simulink model "CPS_heave_noAccelmeter_20221201"  (R2022b)
settings: Solver=ode4  StartTime=0.0  StopTime=sim_time  RelTol=1e-3  EnableMultiTasking=on
values from neighbouring files (symbols this model uses):
  c = 2*dampratio*sqrt(k*M)    [CPS_sims_and_analysis.m]    (also in command_limits_check.m; ringdown-circcyl-M10-d0_001-F1-workspace.mat = 0.125663706144; setup_CPS_parameters.m)
  k = (2*pi*f_nat)^2*M    (= 394.784176044)    [CPS_sims_and_analysis.m]    (also in command_limits_check.m = 98.6960440109; ringdown-circcyl-M10-d0_001-F1-workspace.mat; setup_CPS_parameters.m)
  M = 10    [CPS_sims_and_analysis.m]    (also in command_limits_check.m; ringdown-circcyl-M10-d0_001-F1-workspace.mat; setup_CPS_parameters.m)
  start_position_meters = last_out(6)*-0.03    [CPS_heave_move_2_setpoint.m]
  T = 0.0002    [ringdown-circcyl-M10-d0_001-F1-workspace.mat]    (also in setup_CPS_parameters.m = 0.001)
  Wallace_Cal_tranp = [-0.14949 0.21629 -0.44045 -69.17754 5.14209 66.58631 3.76511 79.12451 -0.93703 -39.93894 -3.18235 -38.82968 ... (36 elements, 6x6)]    [ringdown-circcyl-M10-d0_001-F1-workspace.mat]    (also in setup_CPS_parameters.m = Wallace_Cal')
undefined symbols (not defined in the file or in its folder): DiscIntNeverNeededParam, National_Instruments, PCIe, sigbuilder_block
libraries: sldrtlib x5, dsparch4 x1
settings Model: SimulationMode=external  ExtModeTrigDuration=8000000  Creator=Control Systems  LastModifiedBy=eericks1
settings SolverCC: AlgebraicLoopSolver=TrustRegion
settings DataIOCC: MaxDataPoints=10000  SaveFormat=StructureWithTime  ReturnWorkspaceOutputs=off
settings DebuggingCC: UnconnectedInputMsg=warning  UnconnectedOutputMsg=warning  UnconnectedLineMsg=warning  SFUnexpectedBacktrackingDiag=warning  SFNoUnconditionalDefaultTransitionDiag=warning  SFExecutionAtInitializationDiag=none  SFMachineParentedDataDiag=warning  ArithmeticOperatorsInVariantConditions=warning
settings HardwareCC: ProdBitPerLong=64  ProdHWDeviceType=Intel->x86-64 (Linux 64)  TargetBitPerLong=64  TargetBitPerPointer=64  TargetIntDivRoundTo=Zero  TargetEndianess=LittleEndian  TargetWordSize=64  TargetHWDeviceType=Intel->x86-64
settings ModelReferenceCC: EnableRefExpFcnMdlSchedulingChecks=on  PropagateSignalLabelsOutOfModel=off
settings SFSimCC: SimUseLocalCustomCode=off  CustomCodeUndefinedFunction=UseInterfaceOnly
settings RTWCC: Description=Simulink Desktop Real-Time  SystemTargetFile=sldrt.tlc  TemplateMakefile=sldrt.tmf  RTWUseLocalCustomCode=off  RTWCompilerOptimization=on
settings CodeAppCC: MaxIdLength=95  StateflowObjectComments=on
settings SimulinkDesktopRealTimeCC: TargetLibSuffix=_sldrt.a  TargetPreCompLibLocation=C:\Program Files\MATLAB\R2022b\toolbox\sldrt\lib\win64  TargetLangStandard=C89/C90 (ANSI)  SupportVariableSizeSignals=off
settings ConfigComp: CovMetricSettings=dw  CovSaveCumulativeToWorkspaceVar=on  CovSaveSingleToWorkspaceVar=on  CovExternalEMLEnable=off

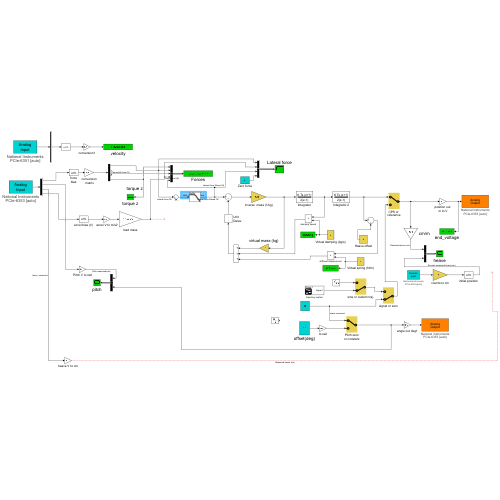
[thumbnail: Simulink's stored preview of the top-level diagram]
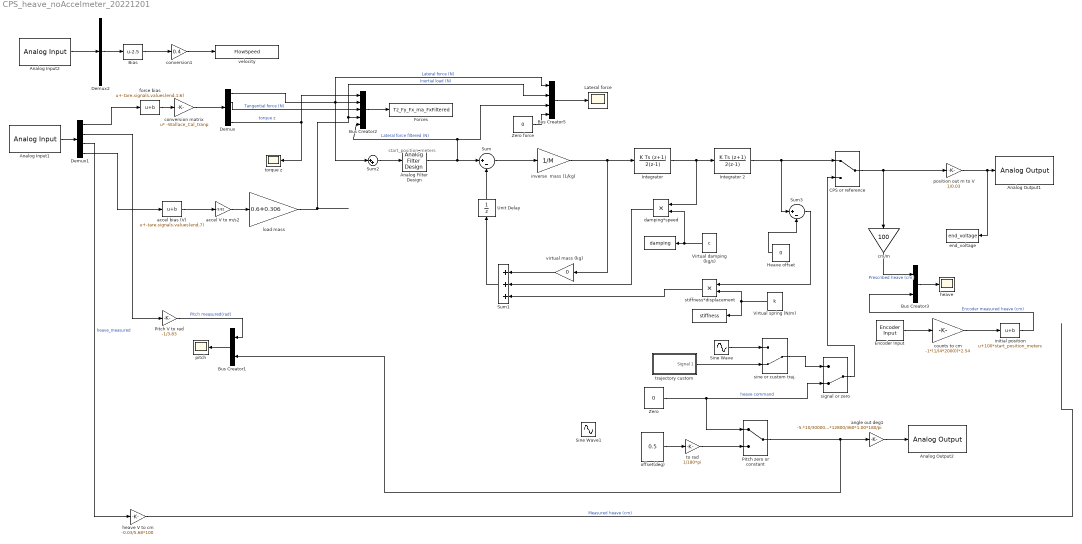
== system CPS_heave_noAccelmeter_20221201 ==
  note: start_position_meters
  " " : ToWorkspace  VariableName=damping  SaveFormat=Structure With Time  SampleTime=-1
  "  " : ToWorkspace  VariableName=stiffness  SaveFormat=Structure With Time  SampleTime=-1
  Analog Filter Design : dsparch4/Analog Filter Design  method=Butterworth  filttype=Lowpass  N=4  Wlo=2*3.14*10  Whi=80  Rp=2  Rs=40
  Analog Input1 : sldrtlib/Analog Input  SampleTime=T  MaxMissedTicks=10  ShowMissedTicks=off  YieldWhenWaiting=off  DrvName=National_Instruments/PCIe-6353  DrvAddress=4294967295  DrvOptions=[0 0 0 2 2 2 2]  Channels=[1: 6 23 24 25]  RangeMode=1  VoltRange=1  DataType=1
      settings: AttributesFormatString=National Instruments\nPCIe-6353 [auto]
  Analog Input2 : sldrtlib/Analog Input  SampleTime=T  MaxMissedTicks=10  ShowMissedTicks=off  YieldWhenWaiting=off  DrvName=National_Instruments/PCIe-6351  DrvAddress=4294967295  DrvOptions=[0 0 0 0 0 0 0]  Channels=[7:10]  RangeMode=1  VoltRange=1  DataType=1
      settings: AttributesFormatString=National Instruments\nPCIe-6351 [auto]
  Analog Output1 : sldrtlib/Analog Output  SampleTime=T  MaxMissedTicks=10  ShowMissedTicks=off  YieldWhenWaiting=off  DrvName=National_Instruments/PCIe-6353  DrvAddress=4294967295  DrvOptions=[0 0 0 2 2 2 2]  Channels=[2]  RangeMode=1  VoltRange=1  InitialValue=[]  FinalValue=[]
      settings: AttributesFormatString=National Instruments\nPCIe-6353 [auto]
  Analog Output2 : sldrtlib/Analog Output  SampleTime=T  MaxMissedTicks=10  ShowMissedTicks=off  YieldWhenWaiting=off  DrvName=National_Instruments/PCIe-6353  DrvAddress=4294967295  DrvOptions=[0 0 0 2 2 2 2]  Channels=[1]  RangeMode=1  VoltRange=1  InitialValue=[]  FinalValue=[]
      settings: AttributesFormatString=National Instruments\nPCIe-6353 [auto]
  Bias : Bias  Bias=-2.5  SaturateOnIntegerOverflow=off
  Bus Creator1 : BusCreator  Inputs=2
  Bus Creator2 : BusCreator  Inputs=5
  Bus Creator3 : BusCreator  Inputs=2
  Bus Creator5 : BusCreator  Inputs=4
  CPS or reference : ManualSwitch
  Demux : Demux  Outputs=[1 1 3 1]
  Demux1 : Demux  Outputs=[6 1 1 1]
  Demux2 : Demux  Outputs=[4]
  Encoder Input : sldrtlib/Encoder Input  SampleTime=T  MaxMissedTicks=10  ShowMissedTicks=off  YieldWhenWaiting=off  DrvName=National_Instruments/PCIe-6353  DrvAddress=4294967295  DrvOptions=[0 0 0 2 2 2 2]  Channels=[1]  QuadMode=3  IndexPulse=1  InputFilter=Inf  DataType=1
      settings: AttributesFormatString=National Instruments\nPCIe-6353 [auto]
  Forces : ToWorkspace  VariableName=Tz_Fy_Fx_ma_FxFiltered  SaveFormat=Structure With Time  SampleTime=-1
  Heave offset : Constant  Value=0  SampleTime=T
  Integrator : DiscreteIntegrator  IntegratorMethod=Integration: Trapezoidal  SampleTime=-1  ICPrevOutput=DiscIntNeverNeededParam  ICPrevScaledInput=DiscIntNeverNeededParam
  Integrator 2 : DiscreteIntegrator  IntegratorMethod=Integration: Trapezoidal  InitialCondition=start_position_meters  SampleTime=-1  ICPrevOutput=DiscIntNeverNeededParam  ICPrevScaledInput=DiscIntNeverNeededParam
  Lateral force : Scope
  Pitch V to rad : Gain  Gain=-1/3.83
  Pitch zero or constant : ManualSwitch
  Sine Wave : Sin  Amplitude=0.05  Frequency=2*3.14*1  SampleTime=0
  Sine Wave1 : Sin  Frequency=2*3.14*0.5  SampleTime=0
  Sum : Sum  Inputs=|+-
  Sum1 : Sum  Inputs=+++
  Sum2 : Sum  Inputs=|++
  Sum3 : Sum  Inputs=|+-
  Unit Delay : UnitDelay  InitialCondition=-start_position_meters*k/M  SampleTime=-1  HasFrameUpgradeWarning=on
  Virtual damping (kg/s) : Constant  Value=c  SampleTime=T
  Virtual spring (N/m) : Constant  Value=k  SampleTime=T
  Zero : Constant  Value=0  SampleTime=T
  Zero force : Constant  Value=0  SampleTime=T
  accel V to m/s2 : Gain  Gain=-9.81
  accel bias (V) : Bias  Bias=-tare.signals.values(end,7)  SaturateOnIntegerOverflow=off
  angle out deg1 : Gain  Gain=-5.*10/30000*12800/360*1.00*180/pi
  cm/m : Gain  Gain=100
  conversion matrix : Gain  Gain=-Wallace_Cal_tranp  Multiplication=Matrix(u*K)
  conversion1 : Gain  Gain=0.4
  counts to cm : Gain  Gain=-1*(1/(4*2000))*2.54
  damping*speed : Product
  end_voltage : ToWorkspace  VariableName=end_voltage  SampleTime=-1
      settings: MaxDataPoints=1
  force bias : Bias  Bias=-tare.signals.values(end,1:6)  SaturateOnIntegerOverflow=off
  heave : Scope
  heave V to cm : Gain  Gain=-0.03/5.68*100
  initial position : Bias  Bias=100*start_position_meters  SaturateOnIntegerOverflow=off
  "inverse  mass (1/kg) " : Gain  Gain=1/M
  load mass : Gain  Gain=0.6+0.306
  offset(deg) : Constant  Value=0.5  SampleTime=T
  pitch : Scope
  position out m to V : Gain  Gain=1/0.03
  signal or zero : ManualSwitch  CurrentSetting=0
  sine or custom traj. : ManualSwitch  CurrentSetting=0
  stiffness*displacement : Product
  to rad : Gain  Gain=1/180*pi
  torque z : Scope
  trajectory custom : Subsystem  Tag=STV Subsys  LoadFcn=sigbuilder_block('load');  StartFcn=sigbuilder_block('start');  StopFcn=sigbuilder_block('stop');  ClipboardFcn=sigbuilder_block('clipboard');  mask(Sigbuilder block){tuvar=[0:10]}
      mask help: Simulink:masks:SigbuilderBlock_MD
      mask init:
      | if ~strcmp(get_param(bdroot(gcbh),'SimulationStatus'),'stopped') tuvar = sigbuilder_block('maskInit'); end
      settings: CopyFcn=sigbuilder_block('copy');  DeleteFcn=sigbuilder_block('delete');  ModelCloseFcn=sigbuilder_block('modelClose');  PreSaveFcn=sigbuilder_block('preSave');  PauseFcn=sigbuilder_block('pause');  ContinueFcn=sigbuilder_block('continue');  NameChangeFcn=sigbuilder_block('namechange');  OpenFcn=sigbuilder_block('open',[270 192.75 550.5 399.75 ]);  CloseFcn=sigbuilder_block('close');
      mask Display: plot(0, 0, 100, 100,[2, 2, 32, 32, 2], [68, 8, 8, 68, 68],[32, 2], [38, 38], [32, 19, 2],[53, 60, 44], [32, 17, 17, 2],[16, 16, 31, 31]);txt = getActiveGroup(gcbh);text(2, 100, txt,'verticalAlignment', 'top');
  velocity : ToWorkspace  VariableName=FlowSpeed  SaveFormat=Structure With Time  SampleTime=-1
  virtual mass (kg) : Gain  Gain=0
  wires:
  Integrator/1 -> damping*speed/1, Integrator 2/1
  "inverse  mass (1/kg) "/1 -> Integrator/1, virtual mass (kg)/1
  Sum/1 -> "inverse  mass (1/kg) "/1
  Sum1/1 -> Unit Delay/1
  Unit Delay/1 -> Sum/2
  damping*speed/1 -> Sum1/2
  virtual mass (kg)/1 -> Sum1/1
  Demux/2 -> Bus Creator2/3  "Tangential force (N)"
  Demux/1 -> Bus Creator5/1, Sum2/1, Bus Creator2/2  "Lateral force (N)"
  force bias/1 -> conversion matrix/1
  Pitch V to rad/1 -> Bus Creator1/1  "Pitch measured(rad)"
  Analog Input1/1 -> Demux1/1
  Demux1/1 -> force bias/1
  Demux1/2 -> Pitch V to rad/1
  heave V to cm/1 -> ?  "Measured heave (cm)"
  Demux1/3 -> heave V to cm/1  "heave_measured"
  Bus Creator1/1 -> pitch/1
  Bus Creator2/1 -> Forces/1
  Zero/1 -> signal or zero/2, Pitch zero or constant/1  "heave command"
  Demux/4 -> torque z/1, Bus Creator2/1  "torque z"
  Pitch zero or constant/1 -> Bus Creator1/2, angle out deg1/1
  angle out deg1/1 -> Analog Output2/1
  to rad/1 -> Pitch zero or constant/2
  offset(deg)/1 -> to rad/1
  conversion1/1 -> velocity/1
  Demux2/1 -> Bias/1
  Bias/1 -> conversion1/1
  Analog Input2/1 -> Demux2/1
  stiffness*displacement/1 -> Sum1/3
  conversion matrix/1 -> Demux/1
  Sine Wave/1 -> sine or custom traj./1
  signal or zero/1 -> CPS or reference/2
  Bus Creator3/1 -> heave/1
  cm/m/1 -> Bus Creator3/1  "Prescribed heave (cm)"
  trajectory custom/1(Signal 1) -> sine or custom traj./2
  sine or custom traj./1 -> signal or zero/1
  Demux1/4 -> accel bias (V)/1
  accel bias (V)/1 -> accel V to m/s2/1
  accel V to m/s2/1 -> load mass/1
  Virtual damping (kg/s)/1 -> damping*speed/2, " "/1
  Virtual spring (N/m)/1 -> "  "/1, stiffness*displacement/2
  load mass/1 -> Bus Creator5/2, Bus Creator2/4  "Inertial load (N)"
  Integrator 2/1 -> CPS or reference/1, Sum3/1
  Heave offset/1 -> Sum3/2
  Sum3/1 -> stiffness*displacement/1
  Bus Creator5/1 -> Lateral force/1
  Zero force/1 -> Bus Creator5/4
  Sum2/1 -> Analog Filter Design/1
  Analog Filter Design/1 -> Sum/1, Bus Creator5/3, Bus Creator2/5  "Lateral force filtered (N)"
  CPS or reference/1 -> position out m to V/1, cm/m/1
  Encoder Input/1 -> counts to cm/1
  counts to cm/1 -> initial position/1
  initial position/1 -> Bus Creator3/2  "Encoder measured heave (cm)"
  position out m to V/1 -> end_voltage/1, Analog Output1/1

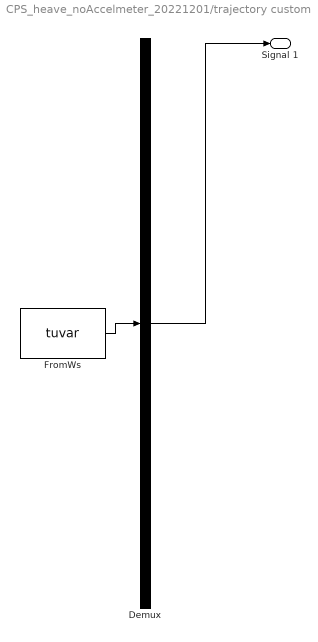
== system CPS_heave_noAccelmeter_20221201/trajectory custom ==
  Demux : Demux  Tag=STV Demux  Outputs=1
      settings: DisplayOption=none
  FromWs : FromWorkspace  Tag=STV FromWs  VariableName=tuvar
      SigBuilderData=|
      | common.afterFinalStr = 'Extrapolate'
      | common.sampleTime = 0
      | dataSet.timeRange = [0 10]
      | dataSet.name = 'Group 1'
      | sbobj.Groups.Name = 'Group 1'
      | sbobj.Groups.Signals.Name = 'Signal 1'
      | sbobj.Groups.Signals.XData = [0 0.0005 0.001 0.0015 0.002 0.0025 0.003 0.0035 0.004 0.0045 0.005 0.0055 ... (1762 elements, 1x1762)]
      | sbobj.Groups.Signals.YData = [0 5.08130081301e-07 2.0325203252e-06 4.57317073171e-06 8.13008130081e-06 1.27032520325e-05 1.82926829268e-05 2.48983739837e-05 3.25203252033e-05 4.11585365854e-05 5.08130081301e-05 6.14837398374e-05 ... (1762 elements, 1x1762)]
  Signal 1 : Outport  Tag=STV Outport
  wires:
  Demux/1 -> Signal 1/1
  FromWs/1 -> Demux/1
